simulink model "modelos"  (R2016a)
settings: Solver=VariableStepAuto  StartTime=0.0  StopTime=100  MaxStep=0.01  RelTol=1e-3
values from neighbouring files (symbols this model uses):
  A = double(subs(jacobian(f),[x1 x2],[0 0]))    [Projeto.m]    (also in q2.m = [0 1  0   0; questao2.m = [0 1 0 0; questao3.m = double(subs(jacobian(f,x),[x1 x2 x3 x4],[0 0 0 0])))
  Am = M    (= 1)    [questao2.m]
  B = double(subs(u, [x1 x2],[0 0]))    [Projeto.m]    (also in q2.m = [  0; questao2.m = [0; 1/M; 0; -1/(M*L)]; questao3.m = double(subs(jacobian(f,u),[x3 x4 u],[0 0 0])))
  Bm = N    [questao2.m]
  C = [1 0 0 ... (first row only)    [Projeto.m]    (also in q2.m = [1 0 0 0]; questao2.m = [1 0 0 0]; questao3.m = [1 0 0 0])
  Cm = eye(3)    [questao2.m]
  Dm = zeros(3,1)    [questao2.m]
  Dsim = zeros(4,1)    [questao2.m]
  K = place(A,B,P1)    [Projeto.m]    (also in questao2.m = kb*T^-1; questao3.m = place(A,B, [pd pd-.01 pd+0.05 pd+0.02]))
  Kl = kd*inv(T)    [questao2.m]
  Km = Ka(:,5:7)    [questao2.m]    (also in questao3.m = Ka(1,5))
  L = Lkf    [Projeto.m]    (also in pendulo_n_linear.m = 1; q2.m = 1; questao2.m = lqr(A',C',V1,q*V2)'; questao3.m = place(A',C',[pd pd-0.05 pd-0.03 pd-0.04])')
  V1 = 0.0001*eye(3)    [Projeto.m]    (also in questao2.m = 0.001*eye(4); questao3.m = 0.001*eye(4))
  x0 = [pi/180*30 0 0]    [Projeto.m]    (also in questao2.m = [0 0 pi/180*10 0]; questao3.m = [0 0 pi/180*20 0])
  x0obs = [pi/180*45 ; 0; 0]    [Projeto.m]    (also in questao2.m = [0 0 pi/180*10 0]; questao3.m = [0; 0; pi/180*20; 0])
libraries: simulink x2
settings Model: Creator=Regner  LastModifiedBy=Regner

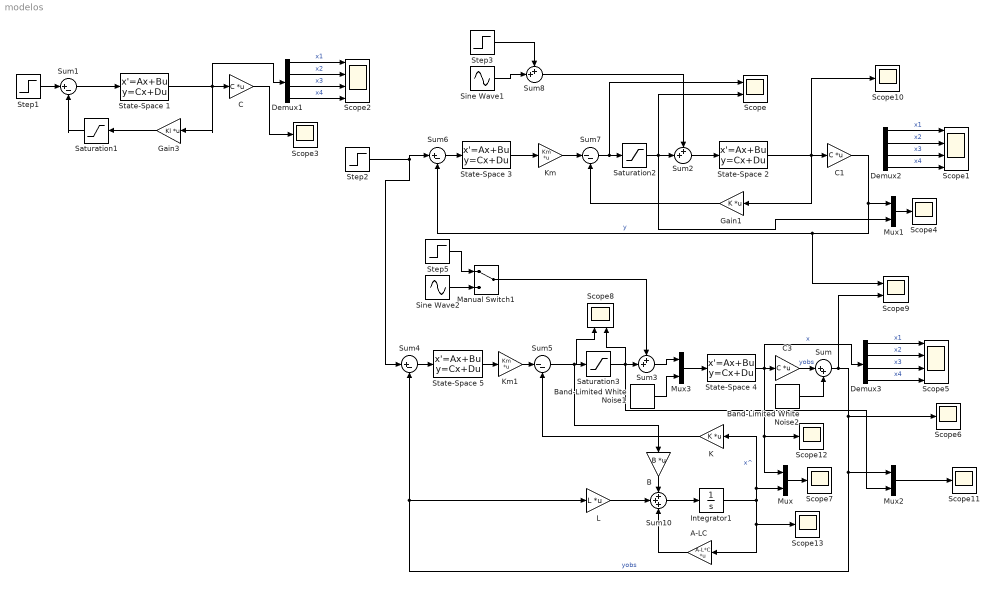
== system modelos ==
  A-LC : Gain  Gain=A-L*C  Multiplication=Matrix(K*u)
  B : Gain  Gain=B  Multiplication=Matrix(K*u)
  Band-Limited White Noise1 : simulink/Sources/Band-Limited White Noise  Cov=diag(V1)  Ts=0.1  seed=[23341]
  Band-Limited White Noise2 : simulink/Sources/Band-Limited White Noise  Cov=V2  Ts=0.1  seed=[23341]
  C : Gain  Gain=C  Multiplication=Matrix(K*u)
  C1 : Gain  Gain=C  Multiplication=Matrix(K*u)
  C3 : Gain  Gain=C  Multiplication=Matrix(K*u)
  Demux1 : Demux
  Demux2 : Demux
  Demux3 : Demux
  Gain1 : Gain  Gain=K  Multiplication=Matrix(K*u)
  Gain3 : Gain  Gain=Kl  Multiplication=Matrix(K*u)
  Integrator1 : Integrator  InitialCondition=x0obs  ZeroCross=off
  K : Gain  Gain=K  Multiplication=Matrix(K*u)
  Km : Gain  Gain=Km  Multiplication=Matrix(K*u)
  Km1 : Gain  Gain=Km  Multiplication=Matrix(K*u)
  L : Gain  Gain=L  Multiplication=Matrix(K*u)
  Manual Switch1 : ManualSwitch
  Mux{,1..3} (4 alike) : Mux  Inputs=2
  Saturation1 : Saturate  UpperLimit=50  LowerLimit=-50
  Saturation2 : Saturate  UpperLimit=50  LowerLimit=-50  ZeroCross=off
  Saturation3 : Saturate  UpperLimit=50  LowerLimit=-50  ZeroCross=off
  Scope : Scope  NumInputPorts=2
  Scope1 : Scope  NumInputPorts=4
  Scope{3..4,6..7,10..13} (8 alike) : Scope
  Scope2 : Scope  NumInputPorts=4
  Scope5 : Scope  NumInputPorts=4
  Scope8 : Scope  NumInputPorts=2
  Scope9 : Scope  NumInputPorts=2
  Sine Wave1 : Sin  Amplitude=5  Frequency=0.1  SampleTime=0
  Sine Wave2 : Sin  Amplitude=10  Frequency=0.1  SampleTime=0
  State-Space 1 : StateSpace  A=A  B=B  C=eye(4)  D=Dsim  X0=x0
  State-Space 2 : StateSpace  A=A  B=B  C=eye(4)  D=Dsim  X0=x0
  State-Space 3 : StateSpace  A=Am  B=Bm  C=Cm  D=Dm  X0=0
  State-Space 4 : StateSpace  A=A  B=[B eye(4)]  C=eye(4)  D=[Dsim zeros(4,4)]  X0=x0
  State-Space 5 : StateSpace  A=Am  B=Bm  C=Cm  D=Dm  X0=0
  Step1 : Step  Time=0  After=0  SampleTime=0
  Step2 : Step  Time=0  After=0  SampleTime=0
  Step3 : Step  Time=20  After=pi/4  SampleTime=0
  Step5 : Step  Time=20  After=pi/4  SampleTime=0
  Sum : Sum  Inputs=|++
  Sum1 : Sum  Inputs=|+-
  Sum10 : Sum  Inputs=+++
  Sum2 : Sum  Inputs=++|
  Sum3 : Sum  Inputs=++|
  Sum4 : Sum  Inputs=|+-
  Sum5 : Sum  Inputs=|--
  Sum6 : Sum  Inputs=|+-
  Sum7 : Sum  Inputs=|--
  Sum8 : Sum  Inputs=++|
  wires:
  Demux1/1 -> Scope2/1  "x1"
  Demux1/2 -> Scope2/2  "x2"
  Demux1/3 -> Scope2/3  "x3"
  Demux1/4 -> Scope2/4  "x4"
  C/1 -> Scope3/1
  State-Space 1/1 -> C/1, Demux1/1, Gain3/1
  Step1/1 -> Sum1/1
  Sum1/1 -> State-Space 1/1
  Gain3/1 -> Saturation1/1
  Saturation1/1 -> Sum1/2
  Demux3/1 -> Scope5/1  "x1"
  Demux3/2 -> Scope5/2  "x2"
  Demux3/3 -> Scope5/3  "x3"
  Demux3/4 -> Scope5/4  "x4"
  State-Space 4/1 -> C3/1, Demux3/1, Scope12/1, Mux/1  "x"
  Step2/1 -> Sum6/1, Sum4/1
  Sum4/1 -> State-Space 5/1
  K/1 -> Sum5/2
  State-Space 5/1 -> Km1/1
  Km1/1 -> Sum5/1
  Mux3/1 -> State-Space 4/1
  Sum5/1 -> Scope8/1, B/1, Saturation3/1
  Demux2/1 -> Scope1/1  "x1"
  Demux2/2 -> Scope1/2  "x2"
  Demux2/3 -> Scope1/3  "x3"
  Demux2/4 -> Scope1/4  "x4"
  C1/1 -> Mux1/1, Scope9/1, Sum6/2  "y"
  State-Space 2/1 -> Scope10/1, Gain1/1, C1/1
  Sum6/1 -> State-Space 3/1
  Gain1/1 -> Sum7/2
  State-Space 3/1 -> Km/1
  Km/1 -> Sum7/1
  Sum2/1 -> State-Space 2/1
  Sum8/1 -> Sum2/1
  Sum7/1 -> Scope/1, Saturation2/1
  Saturation2/1 -> Scope/2, Mux1/2, Sum2/2
  Saturation3/1 -> Scope8/2, Mux2/2, Sum3/2
  Sum/1 -> Scope9/2, Mux2/1, L/1, Sum4/2, Scope6/1  "yobs"
  Sum10/1 -> Integrator1/1
  L/1 -> Sum10/2
  A-LC/1 -> Sum10/3
  Integrator1/1 -> K/1, Mux/2, Scope13/1, A-LC/1  "x^"
  B/1 -> Sum10/1
  Mux/1 -> Scope7/1
  Sine Wave1/1 -> Sum8/2
  Step3/1 -> Sum8/1
  Manual Switch1/1 -> Sum3/1
  Sine Wave2/1 -> Manual Switch1/2
  Step5/1 -> Manual Switch1/1
  Mux1/1 -> Scope4/1
  Mux2/1 -> Scope11/1
  Sum3/1 -> Mux3/1
  Band-Limited White Noise1/1 -> Mux3/2
  C3/1 -> Sum/1  "yobs"
  Band-Limited White Noise2/1 -> Sum/2
